simulink model "old"  (R2022b)
settings: Solver=FixedStepAuto  StartTime=1000  StopTime=1100  FixedStep=0.01  RelTol=1e-3
model workspace (MATLAB code in the model file):
  | A = ...
  |   [1 0.02;
  |    0 1];
  | 
  | B = [0.0002; 0.02];
  | 
  | C = [0 1];
  | 
  | I = ...
  |   [1 0;
  |    0 1];
  | 
  | P0 = ...
  |   [1 0;
  |    0 1];
  | 
  | PotenciaNegativa = -50000;
  | 
  | PotenciaPositiva = 80000;
  | 
  | Q = ...
  |   [10 0;
  |    0 10];
  | 
  | R = 1000;
  | 
  | T = 0.02;
  | 
  | TorqueMaxNegative = -12;
  | 
  | TorqueMaxPositive = 21;
  | 
  | diff_table_F = [0 0.0005 0.0005 0.0006 0.0006 0.0007 0.0008 0.0008 0.0009 ...
  |                 0.0009 0.001 0.0011 0.0011 0.0012 0.0013 0.0014 0.0014 ...
  |                 0.0015 0.0016 0.0017 0.0018 0.0018 0.0019 0.002 0.0021 ...
  |                 0.0022 0.0023 0.0024 0.0025 0.0026 0.0027 0.0027 0.0028 ...
  |                 0.0029 0.0031 0.0032 0.0033 0.0034 0.0035 0.0036 0.0037 ...
  |                 0.0038 0.0039 0.004 0.0042 0.0043 0.0044 0.0045 0.0046 ...
  |                 0.0048 0.0049 0.005 0.0051 0.0053 0.0054 0.0055 0.0057 ...
  |                 0.0058 0.0059 0.0061 0.0062 0.0064 0.0065 0.0067 0.0068 ...
  |                 0.007 0.0071 0.0073 0.0074 0.0076 0.0077 0.0079 0.008 0.0082 ...
  |                 0.0084 0.0085 0.0087 0.0089 0.009 0.0092 0.0094 0.0095];
  | 
  | diff_table_R = [0 0.0023 0.00253 0.00276 0.00299 0.00322 0.00345 0.00368 ...
  |                 0.00391 0.00414 0.00437 0.0046 0.00483 0.00506 0.00529 ...
  |                 0.00552 0.00575 0.00598 0.00621 0.00644 0.00667 0.0069 ...
  |                 0.00713 0.00736 0.00759 0.00782 0.00805 0.00828 0.00851 ...
  |                 0.00874 0.00897 0.0092 0.00943 0.00966 0.00989 0.01012 ...
  |                 0.01035 0.01058 0.01081 0.01104 0.01127 0.0115 0.01173 ...
  |                 0.01196 0.01219 0.01242 0.01265 0.01288 0.01311 0.01334 ...
  |                 0.01357 0.0138 0.01403 0.01426 0.01449 0.01472 0.01495 ...
  |                 0.01518 0.01541 0.01564 0.01587 0.0161 0.01633 0.01656 ...
  |                 0.01679 0.01702 0.01725 0.01748 0.01771 0.01794 0.01817 ...
  |                 0.0184 0.01863 0.01886 0.01909 0.01932 0.01955 0.01978 ...
  |                 0.02001 0.02024 0.02047 0.0207];
  | 
  | diff_table_ext_F = [0 0.0005 0.0005 0.0006 0.0006 0.0007 0.0008 0.0008 ...
  |                     0.0009 0.0009 0.001 0.0011 0.0011 0.0012 0.0013 0.0014 ...
  |                     0.0014 0.0015 0.0016 0.0017 0.0018 0.0018 0.0019 0.002 ...
  |                     0.0021 0.0022 0.0023 0.0024 0.0025 0.0026 0.0027 0.0027 ...
  |                     0.0028 0.0029 0.0031 0.0032 0.0033 0.0034 0.0035 0.0036 ...
  |                     0.0037 0.0038 0.0039 0.004 0.0042 0.0043 0.0044 0.0045 ...
  |                     0.0046 0.0048 0.0049 0.005 0.0051 0.0053 0.0054 0.0055 ...
  |                     0.0057 0.0058 0.0059 0.0061 0.0062 0.0064 0.0065 0.0067 ...
  |                     0.0068 0.007 0.0071 0.0073 0.0074 0.0076 0.0077 0.0079 ...
  |                     0.008 0.0082 0.0084 0.0085 0.0087 0.0089 0.009 0.0092 ...
  |                     0.0094 0.0095 0.0097 0.0099 0.01 0.0102 0.0104 0.0105 ...
  |                     0.0107 0.0109 0.011 0.0112 0.0114 0.0115 0.0117 0.0119 ...
  |                     0.012 0.0122 0.0124 0.0125 0.0127];
  | 
  | diff_table_ext_R = [0 0.0023 0.00253 0.00276 0.00299 0.00322 0.00345 0.00368 ...
  |                     0.00391 0.00414 0.00437 0.0046 0.00483 0.00506 0.00529 ...
  |                     0.00552 0.00575 0.00598 0.00621 0.00644 0.00667 0.0069 ...
  |                     0.00713 0.00736 0.00759 0.00782 0.00805 0.00828 0.00851 ...
  |                     0.00874 0.00897 0.0092 0.00943 0.00966 0.00989 0.01012 ...
  |                     0.01035 0.01058 0.01081 0.01104 0.01127 0.0115 0.01173 ...
  |                     0.01196 0.01219 0.01242 0.01265 0.01288 0.01311 0.01334 ...
  |                     0.01357 0.0138 0.01403 0.01426 0.01449 0.01472 0.01495 ...
  |                     0.01518 0.01541 0.01564 0.01587 0.0161 0.01633 0.01656 ...
  |                     0.01679 0.01702 0.01725 0.01748 0.01771 0.01794 0.01817 ...
  |                     0.0184 0.01863 0.01886 0.01909 0.01932 0.01955 0.01978 ...
  |                     0.02001 0.02024 0.02047 0.0207 0.02093 0.02116 0.02139 ...
  |                     0.02162 0.02185 0.02208 0.02231 0.02254 0.02277 0.023 ...
  |                     0.02323 0.02346 0.02369 0.02392 0.02415 0.02438 0.02461 ...
  |                     0.02484 0.02507];
  | 
  | pdl_threshold = 0.3;
  | 
  | r_torquedis = 0.7;
  | 
  | str_threshold = 1;
libraries: simulink_extras x5, dspfdesign x3, slpidlib x1
(part 1 of 2)
settings Model: Creator=berta  LastModifiedBy=root
settings SolverCC: AlgebraicLoopSolver=TrustRegion
settings DataIOCC: ReturnWorkspaceOutputs=off
settings OptimizationCC: OptimizeBlockIOStorage=off  ReuseModelBlockBuffer=on  EnhancedBackFolding=on  PassReuseOutputArgsThreshold=0  ZeroExternalMemoryAtStartup=off  ZeroInternalMemoryAtStartup=off  OptimizeBlockOrder=speed  DifferentSizesBufferReuse=on
settings DebuggingCC: ParameterTunabilityLossMsg=error  UnconnectedInputMsg=warning  UnconnectedOutputMsg=warning  UnconnectedLineMsg=warning  ArithmeticOperatorsInVariantConditions=warning
settings ModelReferenceCC: EnableRefExpFcnMdlSchedulingChecks=on
settings SFSimCC: MATLABDynamicMemAlloc=off  CustomCodeUndefinedFunction=UseInterfaceOnly
settings RTWCC: Toolchain=Colcon Tools  TargetLang=C++
settings CodeAppCC: ForceParamTrailComments=on  OperatorAnnotations=on  MATLABSourceComments=on
settings GRTTargetCC: TargetLangStandard=C++11 (ISO)  CodeInterfacePackaging=C++ class  MultiInstanceErrorCode=Warning

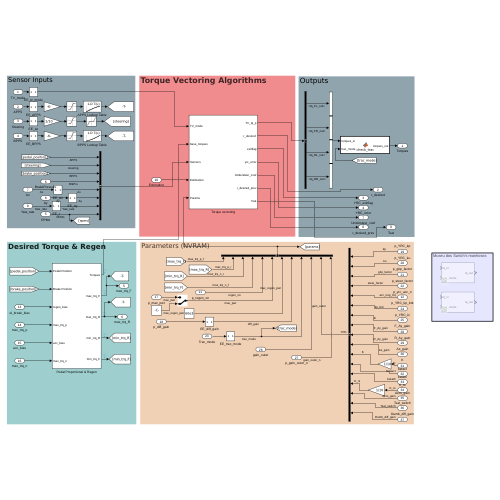
[thumbnail: Simulink's stored preview of the top-level diagram]
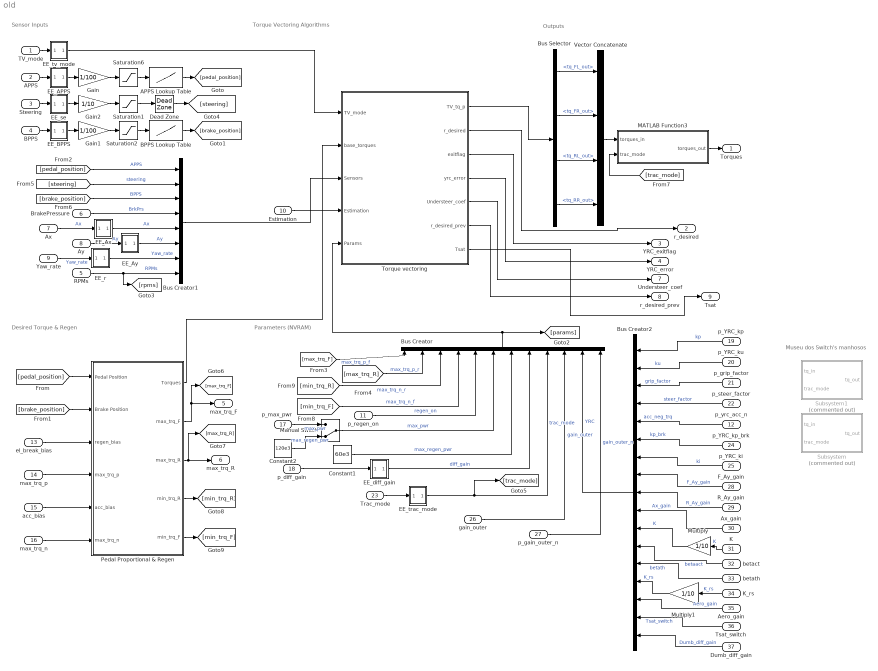
== system old ==
  note: Museu dos Switch's manhosos
  note: Parameters (NVRAM)
  note: Outputs
  note: Torque Vectoring Algorithms
  note: Desired Torque & Regen
  note: Sensor Inputs
  TV_mode : Inport
  APPS : Inport  Port=2
  Steering : Inport  Port=3
  BPPS : Inport  Port=4
  RPMs : Inport  Port=5  PortDimensions=4
  BrakePressure : Inport  Port=6
  Ax : Inport  Port=7
  Ay : Inport  Port=8
  Yaw_rate : Inport  Port=9
  Estimation : Inport  Port=10  PortDimensions=15
  p_regen_on : Inport  Port=11
  p_yrc_acc_n : Inport  Port=12
  el_break_bias : Inport  Port=13
  max_trq_p : Inport  Port=14
  acc_bias : Inport  Port=15
  max_trq_n : Inport  Port=16
  p_max_pwr : Inport  Port=17
  p_diff_gain : Inport  Port=18
  p_YRC_kp : Inport  Port=19
  p_YRC_ku : Inport  Port=20
  p_grip_factor : Inport  Port=21
  p_steer_factor : Inport  Port=22
  Trac_mode : Inport  Port=23
  p_YRC_kp_brk : Inport  Port=24
  p_YRC_ki : Inport  Port=25
  gain_outer : Inport  Port=26
  p_gain_outer_n : Inport  Port=27
  F_Ay_gain : Inport  Port=28
  R_Ay_gain : Inport  Port=29
  Ax_gain : Inport  Port=30
  K : Inport  Port=31
  betact : Inport  Port=32
  betath : Inport  Port=33
  K_rs : Inport  Port=34
  Aero_gain : Inport  Port=35
  Tsat_switch : Inport  Port=36
  Dumb_diff_gain : Inport  Port=37
  APPS Lookup Table : Lookup_n-D  NumberOfTableDimensions=1  BreakpointsForDimension1=[0:0.01:1]  Table=(4*[0:0.01:1])./([0:0.01:1]+3)  InternalRulePriority=Speed  RndMeth=Simplest
  BPPS Lookup Table : Lookup_n-D  NumberOfTableDimensions=1  BreakpointsForDimension1=[0:0.01:1]  Table=-1*(2*[0:0.01:1])./([0:0.01:1]-3)  InternalRulePriority=Speed  RndMeth=Simplest
  Bus Creator : BusCreator  Inputs=12
  Bus Creator1 : BusCreator  Inputs=8
  Bus Creator2 : BusCreator  Inputs=17
  Bus Selector : BusSelector  OutputSignals=tq_FL_out,tq_FR_out,tq_RL_out,tq_RR_out
  Constant1 : Constant  Value=60e3
  Constant2 : Constant  Value=120e3
  Dead Zone : DeadZone  LowerValue=-7  UpperValue=7  LinearizeAsGain=off
  EE_APPS : Subsystem
  EE_Ax : Subsystem
  EE_Ay : Subsystem
  EE_BPPS : Subsystem
  EE_diff_gain : Subsystem
  EE_r : Subsystem
  EE_se : Subsystem
  EE_trac_mode : Subsystem
  EE_tv_mode : Subsystem
  Gain : Gain  Gain=1/100
  Gain1 : Gain  Gain=1/100
  Gain2 : Gain  Gain=1/10
  MATLAB Function3 : MATLAB Function  TreatAsAtomicUnit=on
  Manual Switch : ManualSwitch  CurrentSetting=0
  Multiply : Gain  Gain=1/10
  Multiply1 : Gain  Gain=1/10
  Pedal Proportional & Regen : Subsystem
  Saturation1 : Saturate  UpperLimit=150  LowerLimit=-150  ZeroCross=off
  Saturation2 : Saturate  UpperLimit=1  LowerLimit=0  ZeroCross=off
  Saturation6 : Saturate  UpperLimit=1  LowerLimit=0  ZeroCross=off
  Subsystem : Subsystem  Commented=on
  Subsystem1 : Subsystem  Commented=on
  Torque vectoring : Subsystem
  Vector Concatenate : Concatenate  NumInputs=4
  Torques : Outport
  r_desired : Outport  Port=2
  YRC_exitflag : Outport  Port=3
  YRC_error : Outport  Port=4
  max_trq_F : Outport  Port=5
  max_trq_R : Outport  Port=6
  Understeer_coef : Outport  Port=7
  r_desired_prev : Outport  Port=8
  Tsat : Outport  Port=9
  wires:
  Bus Selector/2 -> Vector Concatenate/2  "<tq_FR_out>"
  Steering/1 -> EE_se/1(In1)
  APPS/1 -> EE_APPS/1(In1)
  Gain/1 -> Saturation6/1
  Gain2/1 -> Saturation1/1
  [pedal_position] -> Pedal Proportional & Regen/1(Pedal Position)
  p_diff_gain/1 -> EE_diff_gain/1(In1)
  el_break_bias/1 -> Pedal Proportional & Regen/3(regen_bias)
  Pedal Proportional & Regen/1(Torques) -> Torque vectoring/2(base_torques)
  Torque vectoring/1(TV_tq_p) -> Bus Selector/1
  Bus Creator/1 -> Torque vectoring/5(Params), [params]
  Gain1/1 -> Saturation2/1
  BPPS/1 -> EE_BPPS/1(In1)
  [brake_position] -> Pedal Proportional & Regen/2(Brake Position)
  TV_mode/1 -> EE_tv_mode/1(In1)
  EE_tv_mode/1(Out1) -> Torque vectoring/1(TV_mode)
  EE_APPS/1(Out1) -> Gain/1
  EE_se/1(Out1) -> Gain2/1
  EE_BPPS/1(Out1) -> Gain1/1
  BrakePressure/1 -> Bus Creator1/4  "BrkPrs"
  Ax/1 -> EE_Ax/1(In1)  "Ax"
  Ay/1 -> EE_Ay/1(In1)  "Ay"
  Yaw_rate/1 -> EE_r/1(In1)  "Yaw_rate"
  Bus Creator1/1 -> Torque vectoring/3(Sensors)
  Saturation1/1 -> Dead Zone/1
  [pedal_position] -> Bus Creator1/1  "APPS"
  [steering] -> Bus Creator1/2  "steering"
  [brake_position] -> Bus Creator1/3  "BPPS"
  Estimation/1 -> Torque vectoring/4(Estimation)
  Constant1/1 -> Bus Creator/7  "max_regen_pwr"
  p_regen_on/1 -> Bus Creator/5  "regen_on"
  p_YRC_kp/1 -> Bus Creator2/1  "kp"
  p_YRC_ku/1 -> Bus Creator2/2  "ku"
  Torque vectoring/2("r_desired ") -> r_desired/1
  RPMs/1 -> [rpms], Bus Creator1/8  "RPMs"
  p_grip_factor/1 -> Bus Creator2/3  "grip_factor"
  p_steer_factor/1 -> Bus Creator2/4  "steer_factor"
  Torque vectoring/3(exitflag) -> YRC_exitflag/1
  EE_diff_gain/1(Out1) -> Bus Creator/8  "diff_gain"
  Bus Selector/1 -> Vector Concatenate/1  "<tq_FL_out>"
  Vector Concatenate/1 -> MATLAB Function3/1(torques_in)
  Bus Selector/3 -> Vector Concatenate/3  "<tq_RL_out>"
  Bus Selector/4 -> Vector Concatenate/4  "<tq_RR_out>"
  Trac_mode/1 -> EE_trac_mode/1(In1)
  EE_trac_mode/1(Out1) -> Bus Creator/9, [trac_mode]  "trac_mode"
  [trac_mode] -> MATLAB Function3/2(trac_mode)
  MATLAB Function3/1(torques_out) -> Torques/1
  [min_trq_F] -> Bus Creator/4  "max_trq_n_f"
  [max_trq_R] -> Bus Creator/2  "max_trq_p_r"
  [max_trq_F] -> Bus Creator/1  "max_trq_p_f"
  p_yrc_acc_n/1 -> Bus Creator2/5  "acc_neg_trq"
  [min_trq_R] -> Bus Creator/3  "max_trq_n_r"
  Saturation6/1 -> APPS Lookup Table/1
  APPS Lookup Table/1 -> [pedal_position]
  Saturation2/1 -> BPPS Lookup Table/1
  BPPS Lookup Table/1 -> [brake_position]
  EE_Ax/1(Out1) -> Bus Creator1/5  "Ax"
  EE_Ay/1(Out1) -> Bus Creator1/6  "Ay"
  EE_r/1(Out1) -> Bus Creator1/7  "Yaw_rate"
  p_YRC_kp_brk/1 -> Bus Creator2/6  "kp_brk"
  p_YRC_ki/1 -> Bus Creator2/7  "ki"
  Torque vectoring/4(yrc_error) -> YRC_error/1
  Bus Creator2/1 -> Bus Creator/11  "YRC"
  gain_outer/1 -> Bus Creator/10  "gain_outer"
  p_gain_outer_n/1 -> Bus Creator/12  "gain_outer_n"
  Pedal Proportional & Regen/2(max_trq_F) -> max_trq_F/1, [max_trq_F]
  Pedal Proportional & Regen/5(min_trq_F) -> [min_trq_F]
  Pedal Proportional & Regen/4(min_trq_R) -> [min_trq_R]
  Pedal Proportional & Regen/3(max_trq_R) -> max_trq_R/1, [max_trq_R]
  max_trq_p/1 -> Pedal Proportional & Regen/4(max_trq_p)
  acc_bias/1 -> Pedal Proportional & Regen/5(acc_bias)
  max_trq_n/1 -> Pedal Proportional & Regen/6(max_trq_n)
  Torque vectoring/5(Understeer_coef) -> Understeer_coef/1
  Constant2/1 -> Manual Switch/2  "max_regen_pwr"
  p_max_pwr/1 -> Manual Switch/1  "max_pwr"
  Manual Switch/1 -> Bus Creator/6  "max_pwr"
  Dead Zone/1 -> [steering]
  F_Ay_gain/1 -> Bus Creator2/8  "F_Ay_gain"
  R_Ay_gain/1 -> Bus Creator2/9  "R_Ay_gain"
  Ax_gain/1 -> Bus Creator2/10  "Ax_gain"
  K/1 -> Multiply/1  "K"
  betath/1 -> Bus Creator2/13  "betath"
  betact/1 -> Bus Creator2/12  "betaact"
  K_rs/1 -> Multiply1/1  "K_rs"
  Multiply/1 -> Bus Creator2/11  "K"
  Multiply1/1 -> Bus Creator2/14  "K_rs"
  Torque vectoring/6(r_desired_prev) -> r_desired_prev/1
  Torque vectoring/7(Tsat) -> Tsat/1
  Aero_gain/1 -> Bus Creator2/15  "Aero_gain"
  Tsat_switch/1 -> Bus Creator2/16  "Tsat_switch"
  Dumb_diff_gain/1 -> Bus Creator2/17  "Dumb_diff_gain"

== system old/EE_APPS ==
  In1 : Inport
  Max : MinMax  Function=max  Inputs=2
  Mode_APPS_overwrite : Constant  Value=0
  Out1 : Outport
  wires:
  In1/1 -> Max/1
  Mode_APPS_overwrite/1 -> Max/2
  Max/1 -> Out1/1

== system old/EE_Ax ==
  In1 : Inport
  Ax_EE_overwrite : Constant  Value=0
  Switch : Switch  Criteria=u2 ~= 0  SaturateOnIntegerOverflow=off  InputSameDT=off
  Out1 : Outport
  wires:
  In1/1 -> Switch/3
  Ax_EE_overwrite/1 -> Switch/1, Switch/2
  Switch/1 -> Out1/1

== system old/EE_Ay ==
  In1 : Inport
  Ay_EE_overwrite : Constant  Value=0
  Switch : Switch  Criteria=u2 ~= 0  SaturateOnIntegerOverflow=off  InputSameDT=off
  Out1 : Outport
  wires:
  In1/1 -> Switch/3
  Ay_EE_overwrite/1 -> Switch/1, Switch/2
  Switch/1 -> Out1/1

== system old/EE_BPPS ==
  In1 : Inport
  BPPS_EE_overwrite : Constant  Value=0
  Max : MinMax  Function=max  Inputs=2
  Out1 : Outport
  wires:
  In1/1 -> Max/1
  BPPS_EE_overwrite/1 -> Max/2
  Max/1 -> Out1/1

== system old/EE_diff_gain ==
  In1 : Inport
  Diff_EE_overwrite : Constant  Value=0
  Max : MinMax  Function=max  Inputs=2
  Out1 : Outport
  wires:
  In1/1 -> Max/1
  Diff_EE_overwrite/1 -> Max/2
  Max/1 -> Out1/1

== system old/EE_r ==
  In1 : Inport
  Switch : Switch  Criteria=u2 ~= 0  SaturateOnIntegerOverflow=off  InputSameDT=off
  r_EE_overwrite : Constant  Value=0
  Out1 : Outport
  wires:
  In1/1 -> Switch/3
  r_EE_overwrite/1 -> Switch/1, Switch/2
  Switch/1 -> Out1/1

== system old/EE_se ==
  In1 : Inport
  Switch : Switch  Criteria=u2 ~= 0  SaturateOnIntegerOverflow=off  InputSameDT=off
  se_EE_overwrite : Constant  Value=0
  Out1 : Outport
  wires:
  In1/1 -> Switch/3
  se_EE_overwrite/1 -> Switch/1, Switch/2
  Switch/1 -> Out1/1

== system old/EE_trac_mode ==
  In1 : Inport
  Max : MinMax  Function=max  Inputs=2
  Mode_Trac_EE_overwrite : Constant  Value=0
  Out1 : Outport
  wires:
  In1/1 -> Max/1
  Mode_Trac_EE_overwrite/1 -> Max/2
  Max/1 -> Out1/1

== system old/EE_tv_mode ==
  In1 : Inport
  Max : MinMax  Function=max  Inputs=2
  Mode_TV_EE_overwrite : Constant  Value=0
  Out1 : Outport
  wires:
  In1/1 -> Max/1
  Mode_TV_EE_overwrite/1 -> Max/2
  Max/1 -> Out1/1

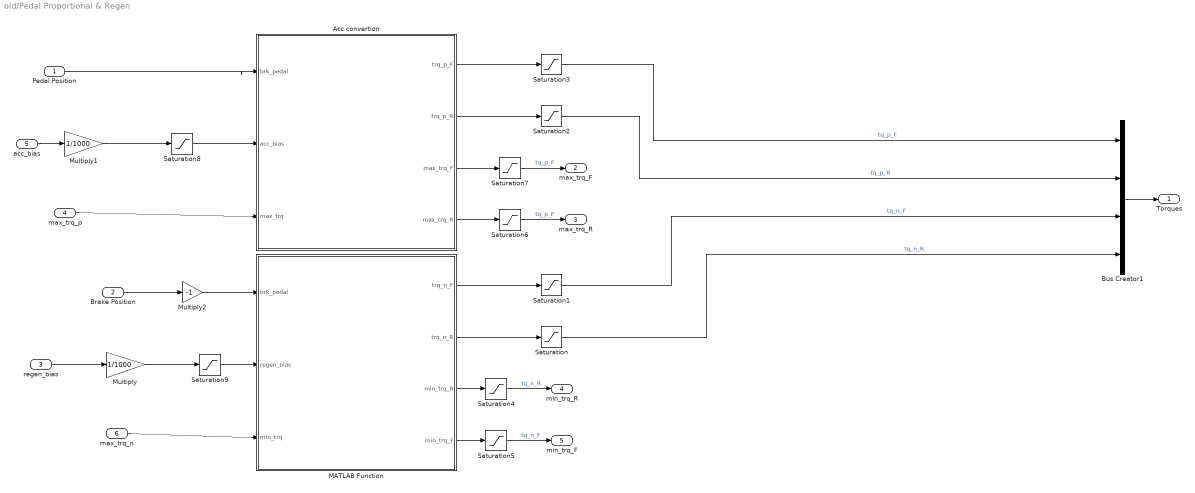
== system old/Pedal Proportional & Regen ==
  Pedal Position : Inport
  Brake Position : Inport  Port=2
  regen_bias : Inport  Port=3
  max_trq_p : Inport  Port=4
  acc_bias : Inport  Port=5
  max_trq_n : Inport  Port=6
  Acc convertion : MATLAB Function  TreatAsAtomicUnit=on
  Bus Creator1 : BusCreator  Inputs=4
  MATLAB Function : MATLAB Function  TreatAsAtomicUnit=on
  Multiply : Gain  Gain=1/1000
  Multiply1 : Gain  Gain=1/1000
  Multiply2 : Gain  Gain=-1
  Saturation : Saturate  UpperLimit=0  LowerLimit=-21000
  Saturation1 : Saturate  UpperLimit=0  LowerLimit=-21000
  Saturation{2..7} (6 alike) : Saturate  UpperLimit=21000  LowerLimit=0
  Saturation8 : Saturate  UpperLimit=1  LowerLimit=0
  Saturation9 : Saturate  UpperLimit=1  LowerLimit=0
  Torques : Outport
  max_trq_F : Outport  Port=2
  max_trq_R : Outport  Port=3
  min_trq_R : Outport  Port=4
  min_trq_F : Outport  Port=5
  wires:
  Bus Creator1/1 -> Torques/1
  Saturation/1 -> Bus Creator1/4  "tq_n_R"
  Saturation1/1 -> Bus Creator1/3  "tq_n_F"
  MATLAB Function/1(trq_n_F) -> Saturation1/1
  MATLAB Function/2(trq_n_R) -> Saturation/1
  max_trq_n/1 -> MATLAB Function/3(min_trq)
  regen_bias/1 -> Multiply/1
  acc_bias/1 -> Multiply1/1
  max_trq_p/1 -> Acc convertion/3(max_trq)
  Acc convertion/1(trq_p_F) -> Saturation3/1
  Pedal Position/1 -> Acc convertion/1(brk_pedal)
  Acc convertion/2(trq_p_R) -> Saturation2/1
  Saturation3/1 -> Bus Creator1/1  "tq_p_F"
  Saturation2/1 -> Bus Creator1/2  "tq_p_R"
  MATLAB Function/3(min_trq_R) -> Saturation4/1
  Saturation4/1 -> min_trq_R/1  "tq_n_R"
  MATLAB Function/4(min_trq_F) -> Saturation5/1
  Saturation5/1 -> min_trq_F/1  "tq_n_F"
  Acc convertion/4(max_trq_R) -> Saturation6/1
  Saturation6/1 -> max_trq_R/1  "tq_p_F"
  Acc convertion/3(max_trq_F) -> Saturation7/1
  Saturation7/1 -> max_trq_F/1  "tq_p_F"
  Multiply2/1 -> MATLAB Function/1(brk_pedal)
  Brake Position/1 -> Multiply2/1
  Multiply1/1 -> Saturation8/1
  Saturation8/1 -> Acc convertion/2(acc_bias)
  Saturation9/1 -> MATLAB Function/2(regen_bias)
  Multiply/1 -> Saturation9/1

== system old/Subsystem ==
  tq_in : Inport
  trac_mode : Inport  Port=2
  Constant : Constant
  Gain : Gain  Gain=0
  Subtract : Sum  Inputs=+-
  Switch : Switch  Criteria=u2 ~= 0  SaturateOnIntegerOverflow=off  InputSameDT=off
  tq_out : Outport
  wires:
  Subtract/1 -> Switch/2
  Switch/1 -> tq_out/1
  tq_in/1 -> Switch/1, Gain/1
  trac_mode/1 -> Subtract/1
  Constant/1 -> Subtract/2
  Gain/1 -> Switch/3

== system old/Subsystem1 ==
  tq_in : Inport
  trac_mode : Inport  Port=2
  Constant : Constant  Value=2
  Gain : Gain  Gain=0
  Subtract : Sum  Inputs=+-
  Switch : Switch  Criteria=u2 ~= 0  SaturateOnIntegerOverflow=off  InputSameDT=off
  tq_out : Outport
  wires:
  Subtract/1 -> Switch/2
  Switch/1 -> tq_out/1
  tq_in/1 -> Switch/1, Gain/1
  trac_mode/1 -> Subtract/1
  Constant/1 -> Subtract/2
  Gain/1 -> Switch/3

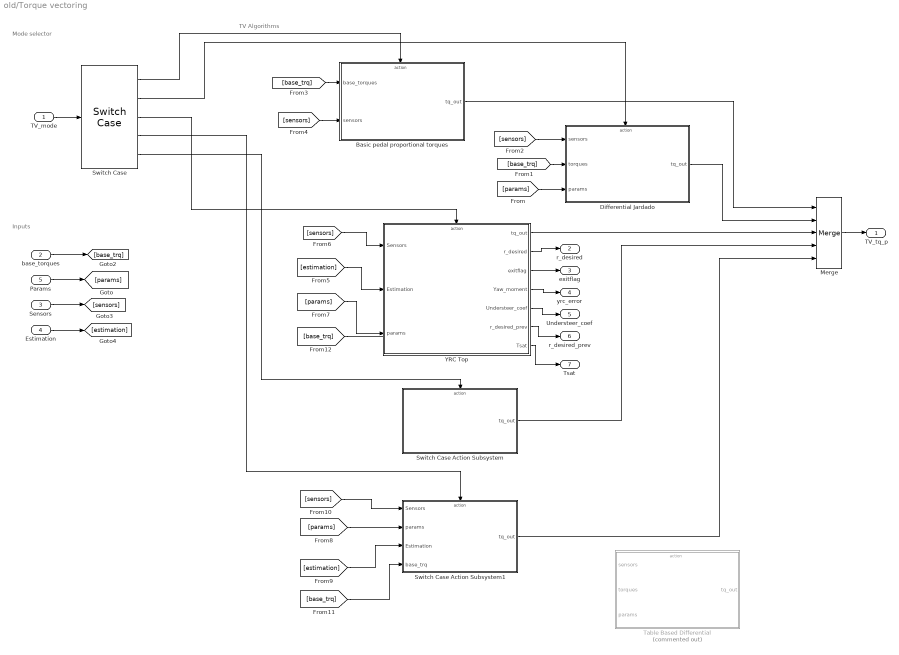
== system old/Torque vectoring ==
  note: Inputs
  note: TV Algorithms
  note: Mode selector
  TV_mode : Inport
  base_torques : Inport  Port=2  PortDimensions=4
  Sensors : Inport  Port=3
  Estimation : Inport  Port=4
  Params : Inport  Port=5
  Basic pedal proportional torques : Subsystem  TreatAsAtomicUnit=on
  Differential Jardado : Subsystem  TreatAsAtomicUnit=on
  Merge : Merge  Inputs=5
  Switch Case : SwitchCase  CaseConditions={1,2,3,4}
  Switch Case Action Subsystem : Subsystem  TreatAsAtomicUnit=on
  Switch Case Action Subsystem1 : Subsystem  TreatAsAtomicUnit=on
  Table Based Differential : Subsystem  Commented=on  TreatAsAtomicUnit=on
  YRC Top : Subsystem  TreatAsAtomicUnit=on
  TV_tq_p : Outport
  "r_desired " : Outport  Port=2
  exitflag : Outport  Port=3
  yrc_error : Outport  Port=4
  Understeer_coef : Outport  Port=5
  r_desired_prev : Outport  Port=6
  Tsat : Outport  Port=7
  wires:
  Merge/1 -> TV_tq_p/1
  Params/1 -> [params]
  TV_mode/1 -> Switch Case/1
  Switch Case/5 -> Switch Case Action Subsystem/Action
  Switch Case/2 -> Differential Jardado/Action
  Switch Case/1 -> Basic pedal proportional torques/Action
  base_torques/1 -> [base_trq]
  [base_trq] -> Differential Jardado/2(torques)
  [base_trq] -> Basic pedal proportional torques/1(base_torques)
  Basic pedal proportional torques/1(tq_out) -> Merge/1
  Differential Jardado/1(tq_out) -> Merge/2
  Switch Case/3 -> YRC Top/Action
  Sensors/1 -> [sensors]
  Estimation/1 -> [estimation]
  [params] -> Differential Jardado/3(params)
  [sensors] -> Differential Jardado/1(sensors)
  YRC Top/1(tq_out) -> Merge/3
  [sensors] -> Basic pedal proportional torques/2(sensors)
  [sensors] -> YRC Top/1(Sensors)
  [estimation] -> YRC Top/2(Estimation)
  [params] -> YRC Top/3(params)
  YRC Top/2("r_desired ") -> "r_desired "/1
  YRC Top/3(exitflag) -> exitflag/1
  Switch Case Action Subsystem/1(tq_out) -> Merge/4
  YRC Top/4(Yaw_moment) -> yrc_error/1
  YRC Top/5(Understeer_coef) -> Understeer_coef/1
  YRC Top/6(r_desired_prev) -> r_desired_prev/1
  YRC Top/7(Tsat) -> Tsat/1
  Switch Case/4 -> Switch Case Action Subsystem1/Action
  Switch Case Action Subsystem1/1(tq_out) -> Merge/5
  [estimation] -> Switch Case Action Subsystem1/3(Estimation)
  [sensors] -> Switch Case Action Subsystem1/1(Sensors)
  [base_trq] -> Switch Case Action Subsystem1/4(base_trq)
  [params] -> Switch Case Action Subsystem1/2(params)
  [base_trq] -> ?

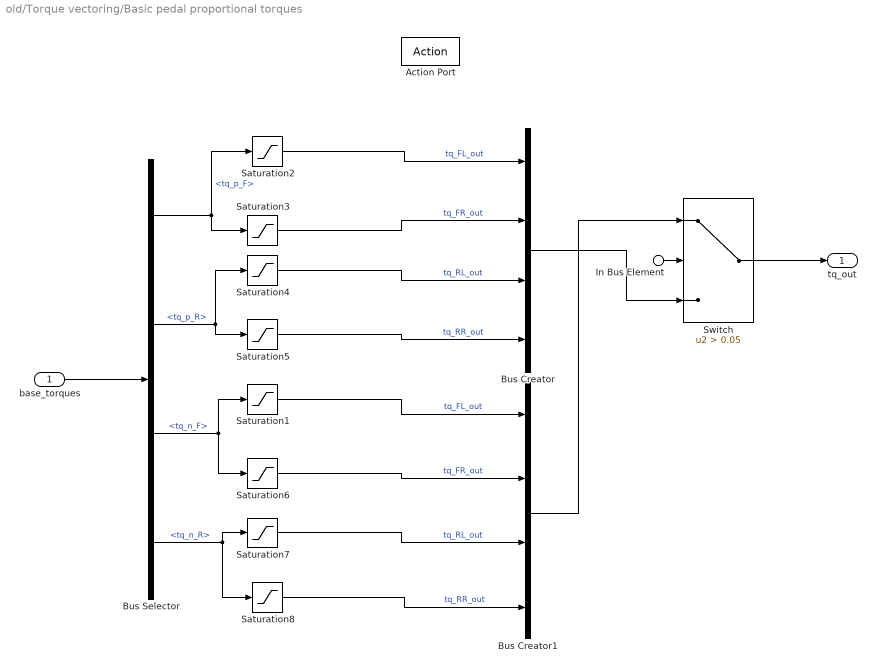
== system old/Torque vectoring/Basic pedal proportional torques ==
  base_torques : Inport
  In Bus Element : Inport  Port=2  PortName=sensors  Element=BPPS
  Action Port : ActionPort  ActionPortLabel=case [ 1 ]:
  Bus Creator : BusCreator  Inputs=4
  Bus Creator1 : BusCreator  Inputs=4
  Bus Selector : BusSelector  OutputSignals=tq_p_F,tq_p_R,tq_n_F,tq_n_R
  Saturation{1,6..8} (4 alike) : Saturate  UpperLimit=0  LowerLimit=-23000  ZeroCross=off
  Saturation{2..5} (4 alike) : Saturate  UpperLimit=21000  LowerLimit=0  ZeroCross=off
  Switch : Switch  Criteria=u2 > Threshold  Threshold=0.05  SaturateOnIntegerOverflow=off  InputSameDT=off
  tq_out : Outport  VectorParamsAs1DForOutWhenUnconnected=off
  wires:
  Saturation5/1 -> Bus Creator/4  "tq_RR_out"
  Saturation4/1 -> Bus Creator/3  "tq_RL_out"
  Bus Selector/1 -> Saturation3/1, Saturation2/1  "<tq_p_F>"
  Bus Selector/2 -> Saturation5/1, Saturation4/1  "<tq_p_R>"
  base_torques/1 -> Bus Selector/1
  Switch/1 -> tq_out/1
  Saturation7/1 -> Bus Creator1/3  "tq_RL_out"
  Saturation8/1 -> Bus Creator1/4  "tq_RR_out"
  Bus Selector/3 -> Saturation6/1, Saturation1/1  "<tq_n_F>"
  Bus Selector/4 -> Saturation7/1, Saturation8/1  "<tq_n_R>"
  In Bus Element/1 -> Switch/2
  Bus Creator/1 -> Switch/3
  Bus Creator1/1 -> Switch/1
  Saturation2/1 -> Bus Creator/1  "tq_FL_out"
  Saturation3/1 -> Bus Creator/2  "tq_FR_out"
  Saturation1/1 -> Bus Creator1/1  "tq_FL_out"
  Saturation6/1 -> Bus Creator1/2  "tq_FR_out"

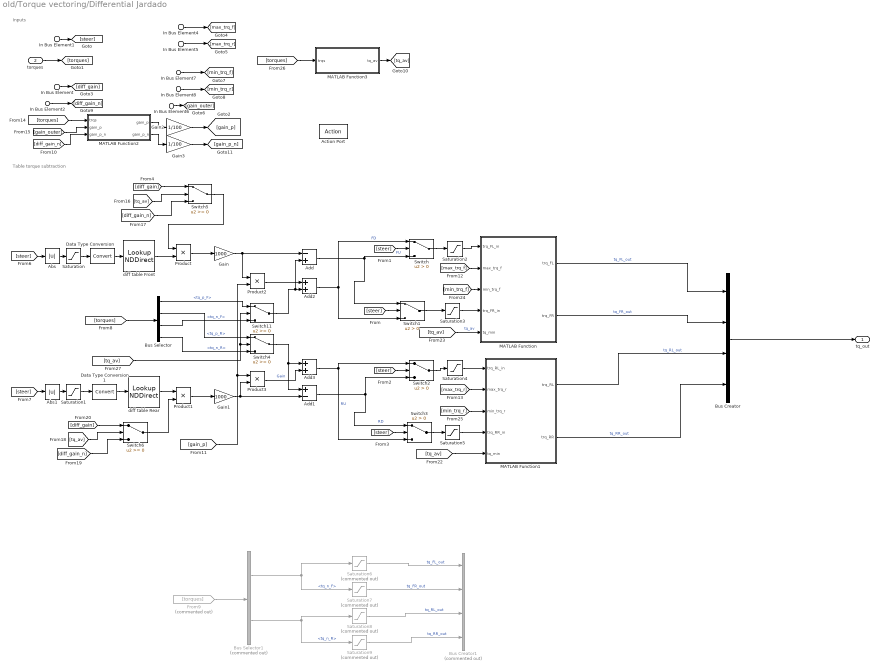
== system old/Torque vectoring/Differential Jardado ==
  note: Inputs
  note: Table torque subtraction
  In Bus Element1 : Inport  PortName=sensors  Element=steering
  torques : Inport  Port=2
  In Bus Element : Inport  Port=3  PortName=params  Element=diff_gain
  In Bus Element4 : Inport  Port=3  PortName=params  Element=max_trq_p_f
  In Bus Element5 : Inport  Port=3  PortName=params  Element=max_trq_p_r
  In Bus Element6 : Inport  Port=3  PortName=params  Element=gain_outer
  In Bus Element7 : Inport  Port=3  PortName=params  Element=max_trq_n_f
  In Bus Element8 : Inport  Port=3  PortName=params  Element=max_trq_n_r
  In Bus Element2 : Inport  Port=3  PortName=params  Element=gain_outer_n
  Action Port : ActionPort  ActionPortLabel=case [ 2 ]:
  Abs : Abs  SaturateOnIntegerOverflow=off
  Abs1 : Abs  SaturateOnIntegerOverflow=off
  Add : Sum  Inputs=-+
  Add1 : Sum  Inputs=+-
  Add2 : Sum
  Add3 : Sum
  Bus Creator : BusCreator  Inputs=4
  Bus Creator1 : BusCreator  Commented=on  Inputs=4
  Bus Selector : BusSelector  OutputSignals=tq_p_F,tq_p_R,tq_n_F,tq_n_R
  Bus Selector1 : BusSelector  Commented=on  OutputSignals=tq_n_F,tq_n_R
  Data Type Conversion : DataTypeConversion  SaturateOnIntegerOverflow=off  RndMeth=Floor
  Data Type Conversion1 : DataTypeConversion  SaturateOnIntegerOverflow=off  RndMeth=Floor
  From9 : From  Commented=on  GotoTag=torques
  Gain : Gain  Gain=1000
  Gain1 : Gain  Gain=1000
  Gain2 : Gain  Gain=1/100
  Gain3 : Gain  Gain=1/100
  MATLAB Function : MATLAB Function  TreatAsAtomicUnit=on
  MATLAB Function1 : MATLAB Function  TreatAsAtomicUnit=on
  MATLAB Function2 : MATLAB Function  TreatAsAtomicUnit=on
  MATLAB Function3 : MATLAB Function  TreatAsAtomicUnit=on
  Product{,1..3} (4 alike) : Product
  Saturation : Saturate  UpperLimit=100  LowerLimit=0  ZeroCross=off
  Saturation1 : Saturate  UpperLimit=100  LowerLimit=0  ZeroCross=off
  Saturation{2..5} (4 alike) : Saturate  UpperLimit=21000  LowerLimit=-21000  ZeroCross=off
  Saturation{6..9} (4 alike) : Saturate  Commented=on  UpperLimit=0  LowerLimit=-21000  ZeroCross=off
  Switch{,1..3} (4 alike) : Switch  Criteria=u2 > Threshold  SaturateOnIntegerOverflow=off  InputSameDT=off
  Switch{4..6,11} (4 alike) : Switch  SaturateOnIntegerOverflow=off  InputSameDT=off
  diff table Front : LookupNDDirect  NumberOfTableDimensions=1  Table=diff_table_ext_F
  diff table Rear : LookupNDDirect  NumberOfTableDimensions=1  Table=diff_table_ext_R
  tq_out : Outport  VectorParamsAs1DForOutWhenUnconnected=off
  wires:
  Bus Selector1/2 -> Saturation8/1, Saturation9/1  "<tq_n_R>"
  Bus Selector1/1 -> Saturation6/1, Saturation7/1  "<tq_n_F>"
  Saturation8/1 -> Bus Creator1/3  "tq_RL_out"
  From9/1 -> Bus Selector1/1
  Saturation6/1 -> Bus Creator1/1  "tq_FL_out"
  Saturation7/1 -> Bus Creator1/2  "tq_FR_out"
  Saturation9/1 -> Bus Creator1/4  "tq_RR_out"
  Bus Creator/1 -> tq_out/1
  MATLAB Function3/1(tq_av) -> [tq_av]
  [torques] -> MATLAB Function3/1(trqs)
  Switch/1 -> Saturation2/1
  Product/1 -> Gain/1
  Gain1/1 -> Add1/2, Product3/2
  [min_trq_r] -> MATLAB Function1/3(min_trq_r)
  [tq_av] -> MATLAB Function/5(tq_min)  "tq_av"
  MATLAB Function/1(trq_FL) -> Bus Creator/1  "tq_FL_out"
  MATLAB Function2/1(gain_p) -> Gain2/1
  [tq_av] -> MATLAB Function1/5(tq_min)
  [min_trq_f] -> MATLAB Function/3(min_trq_f)
  Bus Selector/2 -> Switch4/1  "<tq_p_R>"
  diff table Front/1 -> Product/2
  In Bus Element/1 -> [diff_gain]
  [gain_outer] -> MATLAB Function2/2("gain_p ")
  In Bus Element2/1 -> [diff_gain_n]
  In Bus Element6/1 -> [gain_outer]
  [max_trq_r] -> MATLAB Function1/2(max_trq_r)
  Gain2/1 -> [gain_p]
  In Bus Element4/1 -> [max_trq_f]
  Saturation4/1 -> MATLAB Function1/1(trq_RL_in)
  Saturation5/1 -> MATLAB Function1/4(trq_RR_in)
  MATLAB Function1/1(trq_RL) -> Bus Creator/3  "tq_RL_out"
  [max_trq_f] -> MATLAB Function/2(max_trq_f)
  [torques] -> MATLAB Function2/1(trqs)
  In Bus Element5/1 -> [max_trq_r]
  Add2/1 -> Switch1/3, Switch/1  "FD"
  [steer] -> Switch3/2
  MATLAB Function1/2(trq_RR) -> Bus Creator/4  "tq_RR_out"
  In Bus Element8/1 -> [min_trq_r]
  Data Type Conversion/1 -> diff table Front/1
  Product1/1 -> Gain1/1
  Abs1/1 -> Saturation1/1
  Add3/1 -> Switch3/3, Switch2/1  "RU"
  In Bus Element7/1 -> [min_trq_f]
  Gain/1 -> Add/1, Product2/1
  [torques] -> Bus Selector/1
  Saturation1/1 -> Data Type Conversion1/1
  In Bus Element1/1 -> [steer]
  [steer] -> Abs1/1
  Add1/1 -> Switch2/3, Switch3/1  "RD"
  Saturation/1 -> Data Type Conversion/1
  Switch3/1 -> Saturation5/1
  diff table Rear/1 -> Product1/1
  Data Type Conversion1/1 -> diff table Rear/1
  Abs/1 -> Saturation/1
  Switch2/1 -> Saturation4/1
  [steer] -> Switch1/2
  torques/1 -> [torques]
  [steer] -> Switch2/2
  [steer] -> Switch/2
  Add/1 -> Switch1/1, Switch/3  "FU"
  Bus Selector/1 -> Switch11/1  "<tq_p_F>"
  [steer] -> Abs/1
  Switch1/1 -> Saturation3/1
  Saturation2/1 -> MATLAB Function/1(trq_FL_in)
  Saturation3/1 -> MATLAB Function/4(trq_FR_in)
  MATLAB Function/2(trq_FR) -> Bus Creator/2  "tq_FR_out"
  Switch4/1 -> Add1/1, Add3/1
  Switch11/1 -> Add/2, Add2/2
  [tq_av] -> Switch11/2, Switch4/2
  Bus Selector/3 -> Switch11/3  "<tq_n_F>"
  Bus Selector/4 -> Switch4/3  "<tq_n_R>"
  Product3/1 -> Add3/2  "Gain"
  Product2/1 -> Add2/1
  [gain_p] -> Product2/2, Product3/1
  [tq_av] -> Switch5/2
  [diff_gain_n] -> Switch5/3
  [diff_gain_n] -> MATLAB Function2/3("gain_p_n ")
  Gain3/1 -> [gain_p_n]
  MATLAB Function2/2(gain_p_n) -> Gain3/1
  Switch5/1 -> Product/1
  [diff_gain] -> Switch5/1
  [diff_gain] -> Switch6/1
  [tq_av] -> Switch6/2
  [diff_gain_n] -> Switch6/3
  Switch6/1 -> Product1/2

== system old/Torque vectoring/Switch Case Action Subsystem ==
  Action Port : ActionPort  ActionPortLabel=default:
  Bus Creator : BusCreator  Inputs=4
  Constant{,1..3} (4 alike) : Constant  Value=0
  tq_out : Outport  VectorParamsAs1DForOutWhenUnconnected=off
  wires:
  Constant3/1 -> Bus Creator/4  "tq_RR_out"
  Bus Creator/1 -> tq_out/1
  Constant2/1 -> Bus Creator/3  "tq_RL_out"
  Constant/1 -> Bus Creator/1  "tq_FL_out"
  Constant1/1 -> Bus Creator/2  "tq_FR_out"

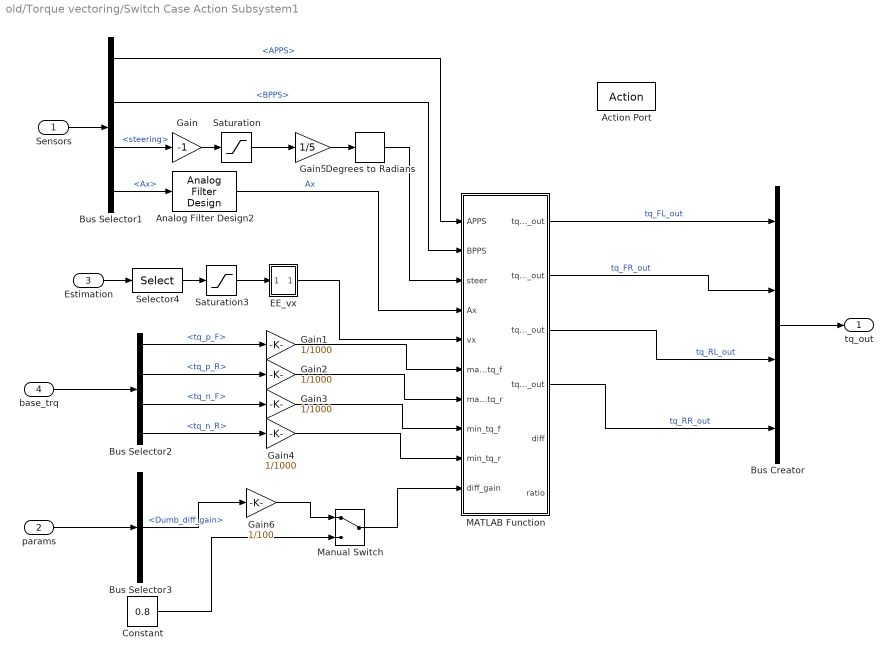
== system old/Torque vectoring/Switch Case Action Subsystem1 ==
  Sensors : Inport
  params : Inport  Port=2
  Estimation : Inport  Port=3
  base_trq : Inport  Port=4
  Action Port : ActionPort  ActionPortLabel=case [ 4 ]:
  Analog Filter Design2 : dspfdesign/Analog Filter Design  method=Chebyshev II  filttype=Lowpass  N=3  Wlo=40  Whi=80  Rp=2  Rs=20
  Bus Creator : BusCreator  Inputs=4
  Bus Selector1 : BusSelector  OutputSignals=APPS,BPPS,steering,Ax
  Bus Selector2 : BusSelector  OutputSignals=tq_p_F,tq_p_R,tq_n_F,tq_n_R
  Bus Selector3 : BusSelector  OutputSignals=YRC.Dumb_diff_gain
  Constant : Constant  Value=0.8
  Degrees to Radians : simulink_extras/Transformations/Degrees to Radians
  EE_vx : Subsystem
  Gain : Gain  Gain=-1
  Gain{1..4} (4 alike) : Gain  Gain=1/1000
  Gain5 : Gain  Gain=1/5
  Gain6 : Gain  Gain=1/100
  MATLAB Function : MATLAB Function  TreatAsAtomicUnit=on
  Manual Switch : ManualSwitch
  Saturation : Saturate  UpperLimit=126  LowerLimit=-126
  Saturation3 : Saturate  UpperLimit=35  LowerLimit=0
  Selector4 : Selector  InputPortWidth=15  IndexOptions=Index vector (dialog)  Indices=[13]  OutputSizes=1
  tq_out : Outport  VectorParamsAs1DForOutWhenUnconnected=off
  wires:
  MATLAB Function/2(tq_FR_out) -> Bus Creator/2  "tq_FR_out"
  Bus Creator/1 -> tq_out/1
  MATLAB Function/3(tq_RL_out) -> Bus Creator/3  "tq_RL_out"
  MATLAB Function/4(tq_RR_out) -> Bus Creator/4  "tq_RR_out"
  Sensors/1 -> Bus Selector1/1
  Bus Selector1/3 -> Gain/1  "<steering>"
  Gain/1 -> Saturation/1
  EE_vx/1(Out1) -> MATLAB Function/5(vx)
  Saturation3/1 -> EE_vx/1(In1)
  Selector4/1 -> Saturation3/1
  Estimation/1 -> Selector4/1
  Bus Selector1/4 -> Analog Filter Design2/1  "<Ax>"
  Analog Filter Design2/1 -> MATLAB Function/4(Ax)  "Ax"
  Bus Selector1/1 -> MATLAB Function/1(APPS)  "<APPS>"
  MATLAB Function/1(tq_FL_out) -> Bus Creator/1  "tq_FL_out"
  Saturation/1 -> Gain5/1
  Gain5/1 -> Degrees to Radians/1
  Degrees to Radians/1 -> MATLAB Function/3(steer)
  Bus Selector2/1 -> Gain1/1  "<tq_p_F>"
  Bus Selector2/2 -> Gain2/1  "<tq_p_R>"
  Bus Selector2/3 -> Gain3/1  "<tq_n_F>"
  Bus Selector2/4 -> Gain4/1  "<tq_n_R>"
  base_trq/1 -> Bus Selector2/1
  Gain1/1 -> MATLAB Function/6(max_tq_f)
  Gain2/1 -> MATLAB Function/7(max_tq_r)
  Gain3/1 -> MATLAB Function/8(min_tq_f)
  Gain4/1 -> MATLAB Function/9(min_tq_r)
  Bus Selector1/2 -> MATLAB Function/2(BPPS)  "<BPPS>"
  params/1 -> Bus Selector3/1
  Constant/1 -> Manual Switch/2
  Manual Switch/1 -> MATLAB Function/10(diff_gain)
  Bus Selector3/1 -> Gain6/1  "<Dumb_diff_gain>"
  Gain6/1 -> Manual Switch/1

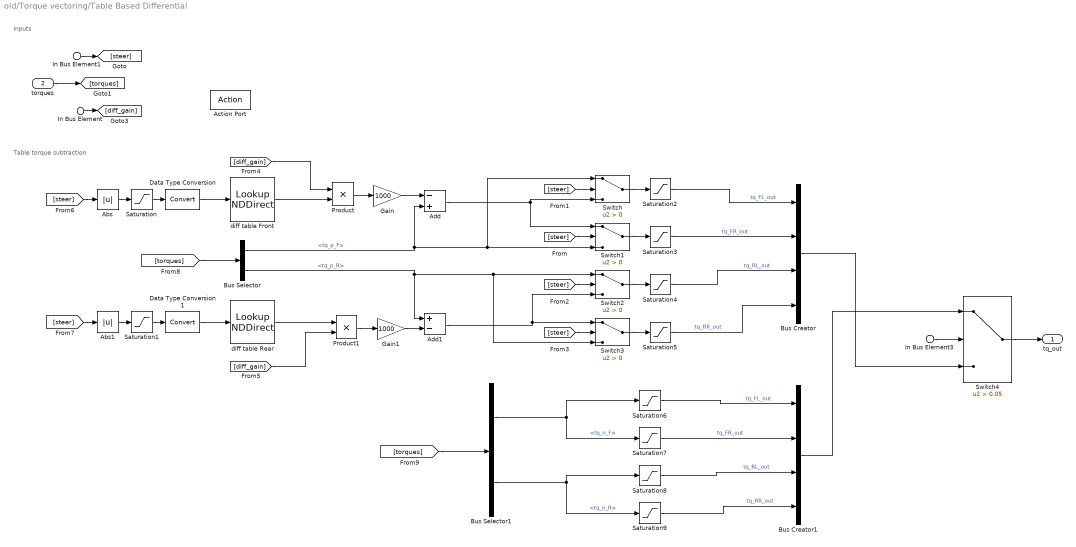
== system old/Torque vectoring/Table Based Differential ==
  note: Inputs
  note: Table torque subtraction
  In Bus Element1 : Inport  PortName=sensors  Element=steering
  In Bus Element3 : Inport  PortName=sensors  Element=BPPS
  torques : Inport  Port=2
  In Bus Element : Inport  Port=3  PortName=params  Element=diff_gain
  Action Port : ActionPort
  Abs : Abs  SaturateOnIntegerOverflow=off
  Abs1 : Abs  SaturateOnIntegerOverflow=off
  Add : Sum  Inputs=-+
  Add1 : Sum  Inputs=+-
  Bus Creator : BusCreator  Inputs=4
  Bus Creator1 : BusCreator  Inputs=4
  Bus Selector : BusSelector  OutputSignals=tq_p_F,tq_p_R
  Bus Selector1 : BusSelector  OutputSignals=tq_n_F,tq_n_R
  Data Type Conversion : DataTypeConversion  SaturateOnIntegerOverflow=off  RndMeth=Floor
  Data Type Conversion1 : DataTypeConversion  SaturateOnIntegerOverflow=off  RndMeth=Floor
  Gain : Gain  Gain=1000
  Gain1 : Gain  Gain=1000
  Product : Product
  Product1 : Product
  Saturation : Saturate  UpperLimit=81  LowerLimit=0  ZeroCross=off
  Saturation1 : Saturate  UpperLimit=81  LowerLimit=0  ZeroCross=off
  Saturation{2..5} (4 alike) : Saturate  UpperLimit=21000  LowerLimit=0  ZeroCross=off
  Saturation{6..9} (4 alike) : Saturate  UpperLimit=0  LowerLimit=-21000  ZeroCross=off
  Switch{,1..3} (4 alike) : Switch  Criteria=u2 > Threshold  SaturateOnIntegerOverflow=off  InputSameDT=off
  Switch4 : Switch  Criteria=u2 > Threshold  Threshold=0.05  SaturateOnIntegerOverflow=off  InputSameDT=off
  diff table Front : LookupNDDirect  NumberOfTableDimensions=1  Table=diff_table_F
  diff table Rear : LookupNDDirect  NumberOfTableDimensions=1  Table=diff_table_R
  tq_out : Outport  VectorParamsAs1DForOutWhenUnconnected=off
  wires:
  [steer] -> Abs/1
  torques/1 -> [torques]
  Saturation5/1 -> Bus Creator/4  "tq_RR_out"
  [steer] -> Abs1/1
  [torques] -> Bus Selector/1
  Saturation1/1 -> Data Type Conversion1/1
  Bus Selector/1 -> Add/2, Switch1/3, Switch/1  "<tq_p_F>"
  [steer] -> Switch/2
  Product1/1 -> Gain1/1
  Add/1 -> Switch1/1, Switch/3
  Saturation4/1 -> Bus Creator/3  "tq_RL_out"
  Saturation/1 -> Data Type Conversion/1
  Bus Selector/2 -> Add1/1, Switch2/1, Switch3/3  "<tq_p_R>"
  [steer] -> Switch3/2
  [steer] -> Switch2/2
  Add1/1 -> Switch2/3, Switch3/1
  Switch/1 -> Saturation2/1
  [steer] -> Switch1/2
  Switch2/1 -> Saturation4/1
  Abs1/1 -> Saturation1/1
  Switch1/1 -> Saturation3/1
  Product/1 -> Gain/1
  In Bus Element/1 -> [diff_gain]
  Switch3/1 -> Saturation5/1
  Abs/1 -> Saturation/1
  In Bus Element1/1 -> [steer]
  Bus Selector1/2 -> Saturation8/1, Saturation9/1  "<tq_n_R>"
  Bus Selector1/1 -> Saturation6/1, Saturation7/1  "<tq_n_F>"
  Saturation8/1 -> Bus Creator1/3  "tq_RL_out"
  [torques] -> Bus Selector1/1
  In Bus Element3/1 -> Switch4/2
  Saturation2/1 -> Bus Creator/1  "tq_FL_out"
  Saturation3/1 -> Bus Creator/2  "tq_FR_out"
  Saturation6/1 -> Bus Creator1/1  "tq_FL_out"
  Saturation7/1 -> Bus Creator1/2  "tq_FR_out"
  Bus Creator/1 -> Switch4/3
  Saturation9/1 -> Bus Creator1/4  "tq_RR_out"
  Bus Creator1/1 -> Switch4/1
  Switch4/1 -> tq_out/1
  [diff_gain] -> Product/1
  [diff_gain] -> Product1/2
  diff table Front/1 -> Product/2
  diff table Rear/1 -> Product1/1
  Data Type Conversion/1 -> diff table Front/1
  Gain/1 -> Add/1
  Gain1/1 -> Add1/2
  Data Type Conversion1/1 -> diff table Rear/1

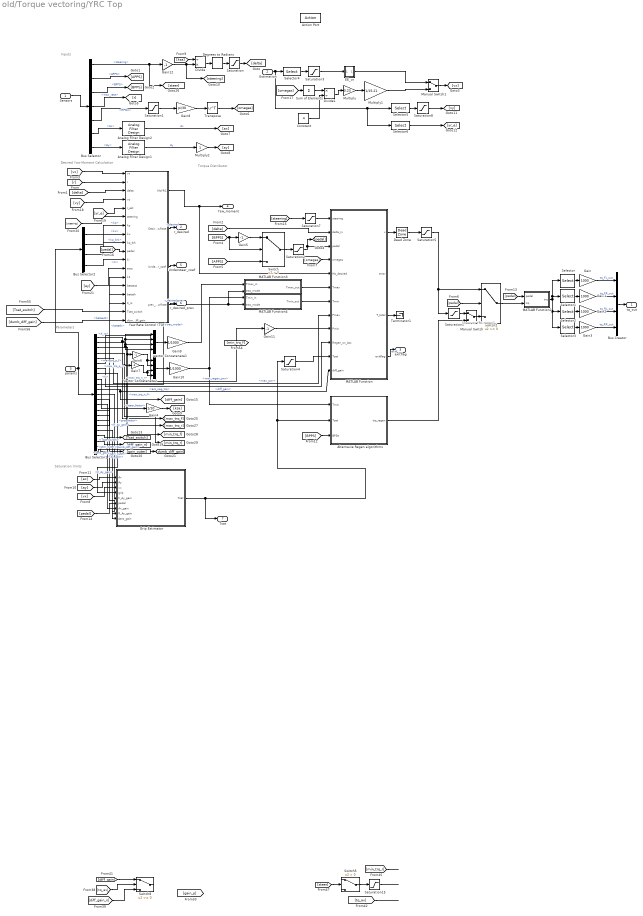
== system old/Torque vectoring/YRC Top ==
  note: linear or
      | YRC regen?
  note: Saturation limits
  note: Parameters
  note: Inputs
  note: Torque Distributor
  note: Desired Yaw Moment Calculation
  Sensors : Inport
  Estimation : Inport  Port=2
  params : Inport  Port=3
  Action Port : ActionPort  ActionPortLabel=case [ 3 ]:
  Alternavie Regen algorithms : Subsystem
  Analog Filter Design1 : dspfdesign/Analog Filter Design  method=Chebyshev II  filttype=Lowpass  N=3  Wlo=40  Whi=80  Rp=2  Rs=20
  Analog Filter Design2 : dspfdesign/Analog Filter Design  method=Chebyshev II  filttype=Lowpass  N=3  Wlo=40  Whi=80  Rp=2  Rs=20
  Bus Creator : BusCreator  Inputs=4
  Bus Selector : BusSelector  OutputSignals=steering,APPS,BPPS,Yaw_rate,RPMs,Ax,Ay
  Bus Selector1 : BusSelector  OutputSignals=max_trq_p_f,max_trq_p_r,max_trq_n_f,max_trq_n_r,max_pwr,max_regen_pwr,YRC.acc_neg_trq,YRC.grip_factor,YRC.steer_factor,trac_mode,diff_gain,YRC.F_Ay_gain,YRC.R_Ay_gain,YRC.Ax_gain,YRC.K,YRC.betaact,YRC.betath,YRC.K_rs,YRC.Aero_gain,YRC.Tsat_switch,gain_outer_n,gain_outer,YRC.Dumb_diff_gain
  Bus Selector2 : BusSelector  OutputSignals=YRC.kp,YRC.ku,YRC.kp_brk,YRC.ki
  Constant : Constant  Value=4
  Dead Zone : DeadZone  LowerValue=-0.01  UpperValue=0.01
  Degrees to Radians : simulink_extras/Transformations/Degrees to Radians
  Divide : Product  Inputs=/*
  Divide1 : Product  Inputs=*/
  EE_vx : Subsystem
  Gain{,1..3} (4 alike) : Gain  Gain=1000
  Gain10 : Gain  Gain=1/1000
  Gain{5..7,11..12} (5 alike) : Gain  Gain=-1
  Gain4 : Gain  Gain=1/10
  Gain8 : Gain  Gain=pi/30
  Gain9 : Gain  Gain=1/1000
  Grip Estimator : Subsystem
  MATLAB Function : MATLAB Function  TreatAsAtomicUnit=on
  MATLAB Function2 : MATLAB Function  TreatAsAtomicUnit=on
  MATLAB Function3 : MATLAB Function  TreatAsAtomicUnit=on
  MATLAB Function4 : MATLAB Function  TreatAsAtomicUnit=on
  Manual Switch : ManualSwitch
  Manual Switch1 : ManualSwitch
  Multiply : Gain  Gain=0.23
  Multiply1 : Gain  Gain=1/15.21
  Multiply2 : Gain
  Saturation : Saturate  UpperLimit=pi/6  LowerLimit=-pi/6
  Saturation1 : Saturate  UpperLimit=30000  LowerLimit=100
  Saturation15 : Saturate  UpperLimit=21000  LowerLimit=-21000  ZeroCross=off
  Saturation2 : Saturate  UpperLimit=1  LowerLimit=-1
  Saturation3 : Saturate  UpperLimit=35  LowerLimit=0
  Saturation4 : Saturate  UpperLimit=21  LowerLimit=2
  Saturation5 : Saturate  UpperLimit=21  LowerLimit=-21
  Saturation6 : Saturate  UpperLimit=0  LowerLimit=-21
  Saturation7 : Saturate  UpperLimit=126  LowerLimit=-126
  Saturation8 : Saturate  UpperLimit=35  LowerLimit=-35
  Selector : Selector  InputPortWidth=4  IndexOptions=Index vector (dialog)  Indices=[1]  OutputSizes=1
  Selector1 : Selector  InputPortWidth=4  IndexOptions=Index vector (dialog)  Indices=[2]  OutputSizes=1
  Selector2 : Selector  InputPortWidth=4  IndexOptions=Index vector (dialog)  Indices=[3]  OutputSizes=1
  Selector3 : Selector  InputPortWidth=4  IndexOptions=Index vector (dialog)  Indices=[4]  OutputSizes=1
  Selector4 : Selector  InputPortWidth=15  IndexOptions=Index vector (dialog)  Indices=[13]  OutputSizes=1
  Selector5 : Selector  InputPortWidth=15  IndexOptions=Index vector (dialog)  Indices=[14]  OutputSizes=1
  Selector6 : Selector  InputPortWidth=15  IndexOptions=Index vector (dialog)  Indices=[15]  OutputSizes=1
  Sum of Elements : Sum  Inputs=+
  Switch : Switch  Criteria=u2 > Threshold  SaturateOnIntegerOverflow=off  InputSameDT=off
  Switch2 : Switch  SaturateOnIntegerOverflow=off  InputSameDT=off
  Switch5 : Switch  Criteria=u2 > Threshold  SaturateOnIntegerOverflow=off  InputSameDT=off
  Switch8 : Switch  SaturateOnIntegerOverflow=off  InputSameDT=off
  Terminator1 : Terminator
  Transpose : Math  Operator=transpose
  Vector Concatenate1 : Concatenate  NumInputs=4
  Vector Concatenate2 : Concatenate  NumInputs=4
  Yaw Rate Control (TOP) : Subsystem
  tq_out : Outport  VectorParamsAs1DForOutWhenUnconnected=off
  "r_desired " : Outport  Port=2
  exitflag : Outport  Port=3
  Yaw_moment : Outport  Port=4
  Understeer_coef : Outport  Port=5
  r_desired_prev : Outport  Port=6
  Tsat : Outport  Port=7
  wires:
  Degrees to Radians/1 -> Saturation/1
  Divide/1 -> Degrees to Radians/1
  [delta] -> MATLAB Function/2(delta_in)
  [BPPS] -> Gain5/1, Switch/2
  Switch/1 -> Saturation2/1
  [delta] -> Yaw Rate Control (TOP)/3(delta)
  Vector Concatenate2/1 -> Gain10/1
  Vector Concatenate1/1 -> Gain9/1
  Yaw Rate Control (TOP)/1("MzYRC ") -> Yaw_moment/1, MATLAB Function/5(Mz_desired)
  Gain5/1 -> Switch/1
  [r] -> Yaw Rate Control (TOP)/2(r)
  [APPS] -> Switch/3
  Sensors/1 -> Bus Selector/1
  Saturation/1 -> [delta]
  Bus Selector/2 -> [APPS]  "<APPS>"
  Bus Selector/3 -> [BPPS]  "<BPPS>"
  Bus Selector/4 -> [r]  "<Yaw_rate>"
  Selector4/1 -> Saturation3/1
  params/1 -> Bus Selector1/1, Bus Selector2/1
  Bus Selector1/2 -> Vector Concatenate1/4, [max_trq_r], Vector Concatenate1/3  "<max_trq_p_r>"
  Bus Selector1/1 -> [max_trq_f], Vector Concatenate1/1, Vector Concatenate1/2  "<max_trq_p_f>"
  Gain6/1 -> Vector Concatenate2/2, Vector Concatenate2/1
  Gain7/1 -> Vector Concatenate2/3, Vector Concatenate2/4
  Bus Selector1/7 -> MATLAB Function/10(Regen_on_Acc)  "<acc_neg_trq>"
  Bus Selector2/1 -> Yaw Rate Control (TOP)/7(kp)  "<kp>"
  Bus Selector2/2 -> Yaw Rate Control (TOP)/8(ku)  "<ku>"
  Yaw Rate Control (TOP)/2(DesiredYawRate) -> "r_desired "/1  "r_desired"
  Bus Selector1/5 -> MATLAB Function/8(Pmax)  "<max_pwr>"
  Bus Selector1/6 -> Gain11/1  "<max_regen_pwr>"
  [omegas] -> MATLAB Function/4(omegas)
  Gain8/1 -> Transpose/1
  Transpose/1 -> [omegas]
  Bus Selector/5 -> Saturation1/1  "<RPMs>"
  Saturation1/1 -> Gain8/1
  Saturation2/1 -> MATLAB Function/3(pedal), [pedal]
  Bus Selector/6 -> Analog Filter Design2/1  "<Ax>"
  [ax] -> Grip Estimator/1(Ax)
  [ay] -> Grip Estimator/2(Ay)
  [vx] -> Grip Estimator/3(vx)
  Gain9/1 -> MATLAB Function3/1(Tmax_in)
  Gain10/1 -> MATLAB Function4/1(Tmin_in), Alternavie Regen algorithms/1(Tmin)
  [ksa] -> Divide/1
  Gain4/1 -> [ksa]
  Bus Selector1/9 -> Gain4/1  "<steer_factor>"
  [pedal] -> Switch2/2
  MATLAB Function/4(exitflag) -> exitflag/1  "exitf"
  [pedal] -> Grip Estimator/6(pedal)
  [BPPS] -> Alternavie Regen algorithms/3(BPSe)
  Saturation4/1 -> MATLAB Function/11(Tsat)
  Gain/1 -> Bus Creator/1  "tq_FL_out"
  Gain1/1 -> Bus Creator/2  "tq_FR_out"
  Bus Creator/1 -> tq_out/1
  Selector3/1 -> Gain3/1
  Selector2/1 -> Gain2/1
  Selector/1 -> Gain/1
  Gain3/1 -> Bus Creator/4  "tq_RR_out"
  Gain2/1 -> Bus Creator/3  "tq_RL_out"
  Selector1/1 -> Gain1/1
  Manual Switch/1 -> Switch2/3
  Alternavie Regen algorithms/1(trq_regen) -> Manual Switch/2
  Saturation5/1 -> Switch2/1, Saturation6/1
  MATLAB Function/1(x) -> Dead Zone/1
  Dead Zone/1 -> Saturation5/1
  Saturation6/1 -> Manual Switch/1
  MATLAB Function2/1(trq) -> Selector2/1, Selector3/1, Selector1/1, Selector/1
  Switch2/1 -> MATLAB Function2/2("trq ")
  [pedal] -> MATLAB Function2/1(pedal)
  Bus Selector1/8 -> Grip Estimator/4(grip)  "<grip_factor>"
  MATLAB Function3/1(Tmax_out) -> MATLAB Function/6(Tmax)
  Bus Selector1/10 -> MATLAB Function3/2(trac_mode), MATLAB Function4/2(trac_mode)  "<trac_mode>"
  MATLAB Function4/1(Tmin_out) -> MATLAB Function/7(Tmin)
  Gain11/1 -> MATLAB Function/9(Pmin)
  [steering] -> Saturation7/1
  Bus Selector1/11 -> [diff_gain], MATLAB Function/12(diff_gain)  "<diff_gain>"
  [vx] -> Yaw Rate Control (TOP)/1(vx)
  Saturation3/1 -> EE_vx/1(In1)
  EE_vx/1(Out1) -> Manual Switch1/1
  Bus Selector1/3 -> [min_trq_f], Gain6/1  "<max_trq_n_f>"
  Bus Selector1/4 -> [min_trq_r], Gain7/1  "<max_trq_n_r>"
  Saturation7/1 -> MATLAB Function/1(steering)
  Bus Selector2/3 -> Yaw Rate Control (TOP)/9(kp_brk)  "<kp_brk>"
  [pedal] -> Yaw Rate Control (TOP)/10(pedal)
  Bus Selector2/4 -> Yaw Rate Control (TOP)/11(ki)  "<ki>"
  MATLAB Function/3(T_total) -> Terminator1/1
  Gain12/1 -> Divide/2, [steering]
  Manual Switch1/1 -> [vx]
  [omegas] -> Sum of Elements/1
  Sum of Elements/1 -> Divide1/1
  Constant/1 -> Divide1/2
  Divide1/1 -> Multiply/1
  Multiply/1 -> Multiply1/1
  Multiply1/1 -> Manual Switch1/2
  Yaw Rate Control (TOP)/3(Understeer_coef) -> Understeer_coef/1
  Bus Selector1/12 -> Grip Estimator/5(F_Ay_gain)  "<F_Ay_gain>"
  Bus Selector1/13 -> Grip Estimator/8(R_Ay_gain)  "<R_Ay_gain>"
  Bus Selector1/14 -> Grip Estimator/7(Ax_gain)  "<Ax_gain>"
  Estimation/1 -> Selector6/1, Selector5/1, Selector4/1
  Selector5/1 -> Saturation8/1
  Saturation8/1 -> [vy]
  Selector6/1 -> [yr_e]
  [vy] -> Yaw Rate Control (TOP)/4(vy)
  [yr_e] -> Yaw Rate Control (TOP)/5(r_est)
  [steering] -> Yaw Rate Control (TOP)/6(steering)
  Analog Filter Design1/1 -> Multiply2/1  "Ay"
  Bus Selector/7 -> Analog Filter Design1/1  "<Ay>"
  Analog Filter Design2/1 -> [ax]  "Ax"
  [ay] -> Yaw Rate Control (TOP)/12(accy)
  Bus Selector1/15 -> Yaw Rate Control (TOP)/13(k1)  "<K>"
  Bus Selector1/16 -> Yaw Rate Control (TOP)/14(betaact)  "<betaact>"
  Bus Selector1/17 -> Yaw Rate Control (TOP)/15(betath)  "<betath>"
  Bus Selector1/18 -> Yaw Rate Control (TOP)/16(K_rs)  "<K_rs>"
  Yaw Rate Control (TOP)/4(prev_desiredYawRate) -> r_desired_prev/1  "r_desired_prev"
  Bus Selector/1 -> [steer], Gain12/1  "<steering>"
  Multiply2/1 -> [ay]
  Bus Selector1/19 -> Grip Estimator/9(Aero_gain)  "<Aero_gain>"
  Grip Estimator/1(Tsat) -> Alternavie Regen algorithms/2(Tsat), Saturation4/1, Tsat/1
  Bus Selector1/20 -> [Tsat_switch]  "<Tsat_switch>"
  Bus Selector1/21 -> [diff_gain_n]  "<gain_outer_n>"
  Bus Selector1/22 -> [gain_outer]  "<gain_outer>"
  [diff_gain_n] -> Switch8/3
  Switch5/1 -> Saturation15/1
  [min_trq_r] -> ?
  [steer] -> Switch5/2
  [tq_av] -> Switch8/2
  Saturation15/1 -> ?
  [tq_av] -> ?
  [diff_gain] -> Switch8/1
  Bus Selector1/23 -> [dumb_diff_gain]  "<Dumb_diff_gain>"
  [Tsat_switch] -> Yaw Rate Control (TOP)/17(Tsat_switch)
  [dumb_diff_gain] -> Yaw Rate Control (TOP)/18(dumb_diff_gain)

== system old/Torque vectoring/Switch Case Action Subsystem1/EE_vx ==
  In1 : Inport
  Max : MinMax  Function=max  Inputs=2
  Vx_EE_overwrite : Constant  Value=0
  Out1 : Outport
  wires:
  In1/1 -> Max/1
  Vx_EE_overwrite/1 -> Max/2
  Max/1 -> Out1/1

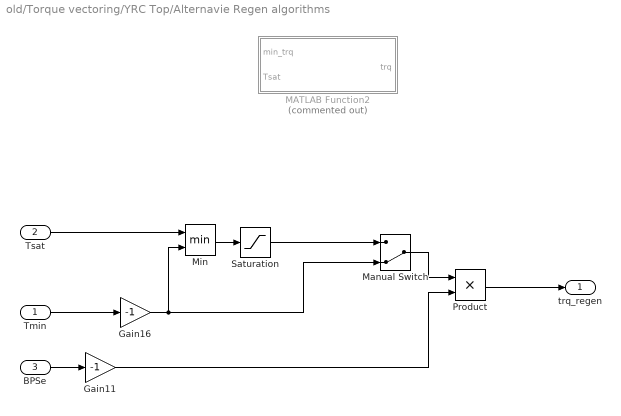
== system old/Torque vectoring/YRC Top/Alternavie Regen algorithms ==
  Tmin : Inport
  Tsat : Inport  Port=2
  BPSe : Inport  Port=3
  Gain11 : Gain  Gain=-1
  Gain16 : Gain  Gain=-1
  MATLAB Function2 : MATLAB Function  Commented=on  TreatAsAtomicUnit=on
  Manual Switch : ManualSwitch  CurrentSetting=0
  Min : MinMax  Inputs=2
  Product : Product
  Saturation : Saturate  UpperLimit=21  LowerLimit=0
  trq_regen : Outport
  wires:
  Gain11/1 -> Product/2
  BPSe/1 -> Gain11/1
  Tmin/1 -> Gain16/1
  Gain16/1 -> Manual Switch/2, Min/2
  Manual Switch/1 -> Product/1
  Tsat/1 -> Min/1
  Min/1 -> Saturation/1
  Saturation/1 -> Manual Switch/1
  Product/1 -> trq_regen/1

== system old/Torque vectoring/YRC Top/EE_vx ==
  In1 : Inport
  Max : MinMax  Function=max  Inputs=2
  Vx_EE_overwrite : Constant  Value=0
  Out1 : Outport
  wires:
  In1/1 -> Max/1
  Vx_EE_overwrite/1 -> Max/2
  Max/1 -> Out1/1

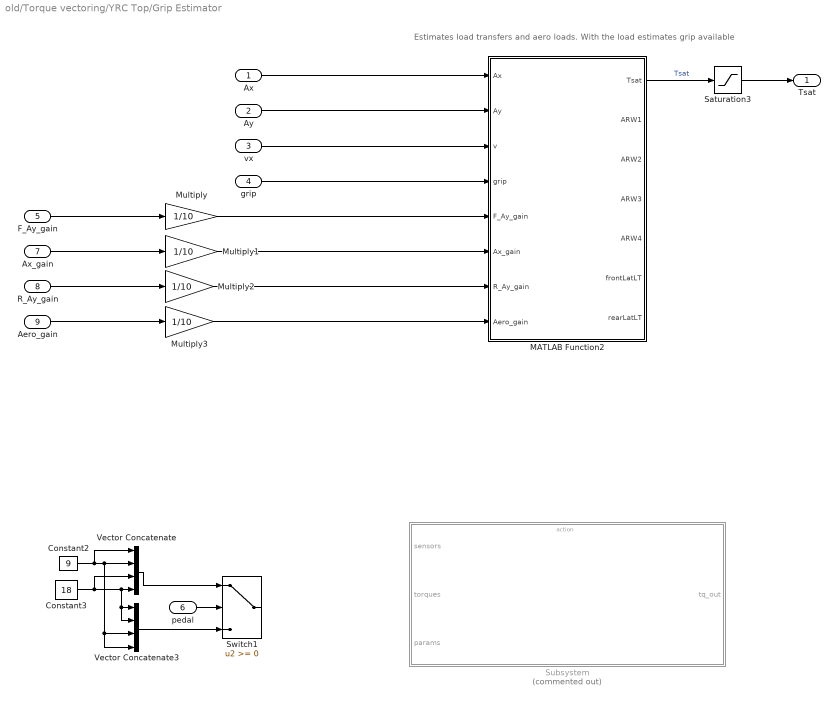
== system old/Torque vectoring/YRC Top/Grip Estimator ==
  note: Estimates load transfers and aero loads. With the load estimates grip available
  Ax : Inport
  Ay : Inport  Port=2
  vx : Inport  Port=3
  grip : Inport  Port=4
  F_Ay_gain : Inport  Port=5
  pedal : Inport  Port=6
  Ax_gain : Inport  Port=7
  R_Ay_gain : Inport  Port=8
  Aero_gain : Inport  Port=9
  Constant2 : Constant  Value=9
  Constant3 : Constant  Value=18
  MATLAB Function2 : MATLAB Function  TreatAsAtomicUnit=on
  Multiply{,1..3} (4 alike) : Gain  Gain=1/10
  Saturation3 : Saturate  UpperLimit=21  LowerLimit=0
  Subsystem : Subsystem  Commented=on
  Switch1 : Switch  SaturateOnIntegerOverflow=off  InputSameDT=off
  Vector Concatenate : Concatenate  NumInputs=4
  Vector Concatenate3 : Concatenate  NumInputs=4
  Tsat : Outport
  wires:
  grip/1 -> MATLAB Function2/4(grip)
  vx/1 -> MATLAB Function2/3(v)
  Saturation3/1 -> Tsat/1
  pedal/1 -> Switch1/2
  Vector Concatenate3/1 -> Switch1/3
  Vector Concatenate/1 -> Switch1/1
  Constant2/1 -> Vector Concatenate/1, Vector Concatenate3/4, Vector Concatenate3/3, Vector Concatenate/2
  Constant3/1 -> Vector Concatenate3/2, Vector Concatenate3/1, Vector Concatenate/4, Vector Concatenate/3
  Multiply/1 -> MATLAB Function2/5(F_Ay_gain)
  F_Ay_gain/1 -> Multiply/1
  Ax_gain/1 -> Multiply1/1
  Multiply1/1 -> MATLAB Function2/6(Ax_gain)
  R_Ay_gain/1 -> Multiply2/1
  Multiply2/1 -> MATLAB Function2/7(R_Ay_gain)
  Ax/1 -> MATLAB Function2/1(Ax)
  Ay/1 -> MATLAB Function2/2(Ay)
  Aero_gain/1 -> Multiply3/1
  Multiply3/1 -> MATLAB Function2/8(Aero_gain)
  MATLAB Function2/1(Tsat) -> Saturation3/1  "Tsat"
